simulink model "UnlinearTest"  (R2016b)
settings: Solver=VariableStepAuto  StartTime=0.0  StopTime=10.0  RelTol=1e-3
settings Model: Creator=lenovo  LastModifiedBy=lenovo

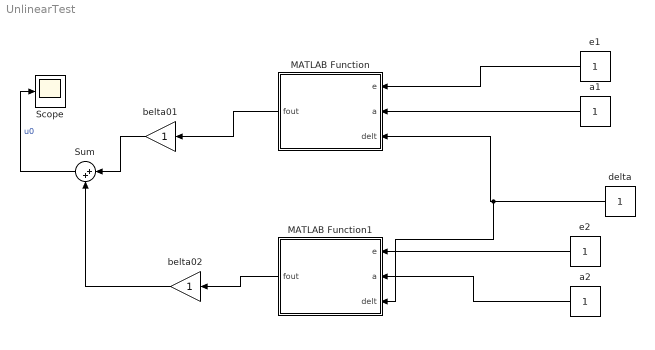
== system UnlinearTest ==
  MATLAB Function : MATLAB Function  TreatAsAtomicUnit=on
  MATLAB Function1 : MATLAB Function  TreatAsAtomicUnit=on
  Scope : Scope
  Sum : Sum  Inputs=|++
  a1 : Constant
  a2 : Constant
  belta01 : Gain
  belta02 : Gain
  delta : Constant
  e1 : Constant
  e2 : Constant
  wires:
  e1/1 -> MATLAB Function/1(e)
  a1/1 -> MATLAB Function/2(a)
  delta/1 -> MATLAB Function1/3(delt), MATLAB Function/3(delt)
  e2/1 -> MATLAB Function1/1(e)
  a2/1 -> MATLAB Function1/2(a)
  MATLAB Function/1(fout) -> belta01/1
  MATLAB Function1/1(fout) -> belta02/1
  belta01/1 -> Sum/1
  belta02/1 -> Sum/2
  Sum/1 -> Scope/1  "u0"

== matlab function UnlinearTest/MATLAB Function1 ==
  data: e input; fout output; a input; delt input
function fout= falfcn(e,a,delt)
if abs(e)>delt
    fal=(abs(e))^a*sign(e);
else
    fal=delt^(1-a);
    fal=e/fal;
end
fout=fal;

end

== matlab function UnlinearTest/MATLAB Function ==
  data: e input; fout output; a input; delt input
function fout= falfcn(e,a,delt)
if abs(e)>delt
    fal=(abs(e))^a*sign(e);
else
    fal=delt^(1-a);
    fal=e/fal;
end
fout=fal;

end
